simulink model "pid_variable"  (R2018a)
settings: Solver=VariableStepAuto  StartTime=0.0  StopTime=10.0  RelTol=1e-3
settings Model: Creator=gonzalo  LastModifiedBy=gonzalo

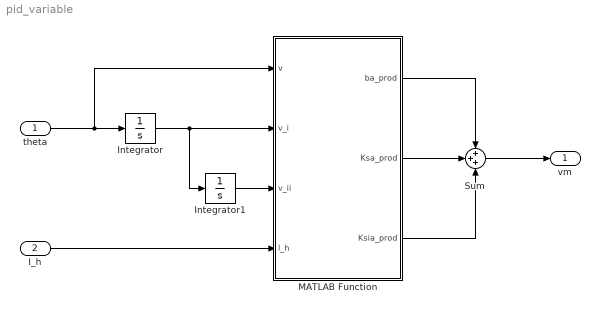
== system pid_variable ==
  theta : Inport
  I_h : Inport  Port=2
  Integrator : Integrator
  Integrator1 : Integrator
  MATLAB Function : MATLAB Function  TreatAsAtomicUnit=on
  Sum : Sum  Inputs=+++
  vm : Outport
  wires:
  theta/1 -> Integrator/1, MATLAB Function/1(v)
  Integrator/1 -> Integrator1/1, MATLAB Function/2(v_i)
  Integrator1/1 -> MATLAB Function/3(v_ii)
  MATLAB Function/2(Ksa_prod) -> Sum/2
  MATLAB Function/3(Ksia_prod) -> Sum/3
  MATLAB Function/1(ba_prod) -> Sum/1
  Sum/1 -> vm/1
  I_h/1 -> MATLAB Function/4(l_h)

== matlab function pid_variable/MATLAB Function ==
  data: ba_prod output; Ksa_prod output; Ksia_prod output; v input; v_i input; v_ii input; l_h input
function [ba_prod, Ksa_prod, Ksia_prod] = fcn(v, v_i, v_ii, l_h)

n = 2.5;
w_pos = 800;

k = 7;

G_s = tf([-(m_c + m_l) 0],[(M_t + m_l) * l_h 0 M_t]);
poles = roots(G.den{1});



ba = 
Ksa =
Ksia = 


ba_prod = ba * v;
Ksa_prod = Ksa * v_i;
Ksia_prod = Ksia * v_ii;



end
